simulink model "TP_EBS_CHERIF"  (R2024b)
settings: Solver=ode45  StartTime=0.0  StopTime=10  RelTol=1e-3
InitFcn:
  | Cte_TP_ABS_CHERIF
values from neighbouring files (symbols this model uses):
  d_arriere = 1.5    [Cte_TP_ABS_CHERIF.m]
  d_avant = 1.5    [Cte_TP_ABS_CHERIF.m]
  f = 0.8    [Cte_TP_ABS_CHERIF.m]
  g = 9.81    [Cte_TP_ABS_CHERIF.m]    (also in Cte_Traction.m)
  h = 0.7    [Cte_TP_ABS_CHERIF.m]
  J = 0.5    [Cte_TP_ABS_CHERIF.m]    (also in Cte_Traction.m)
  Kd = 0    [Cte_TP_ABS_CHERIF.m]
  Ki = 10    [Cte_TP_ABS_CHERIF.m]
  Kp = 100    [Cte_TP_ABS_CHERIF.m]
  L = d_avant + d_arriere    (= 3)    [Cte_TP_ABS_CHERIF.m]    (also in Cte_Traction.m = 0.0005)
  m = 1000    [Cte_TP_ABS_CHERIF.m]    (also in Cte_Traction.m = 1500)
  rRoue = 0.3    [Cte_TP_ABS_CHERIF.m]
  Ts = 0,0001    [Cte_TP_ABS_CHERIF.m]
  v0 = 27.77    [Cte_TP_ABS_CHERIF.m]
undefined symbols (not defined in the file or in its folder): DiscIntNeverNeededParam
libraries: simulink x1
settings Model: Creator=enzoc  LastModifiedBy=enzoc
settings SolverCC: ZeroCrossAlgorithm=Adaptive
settings DebuggingCC: AlgebraicLoopMsg=none  IgnoredZcDiagnostic=none

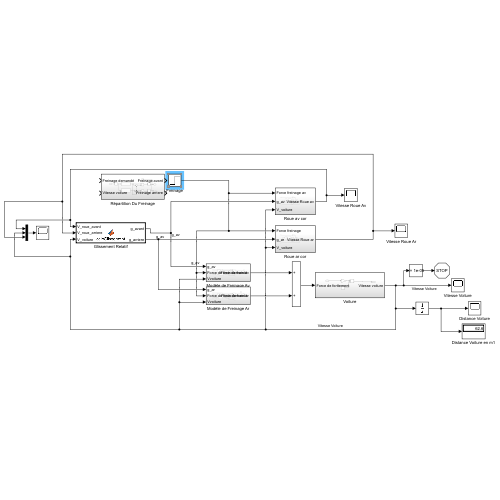
[thumbnail: Simulink's stored preview of the top-level diagram]
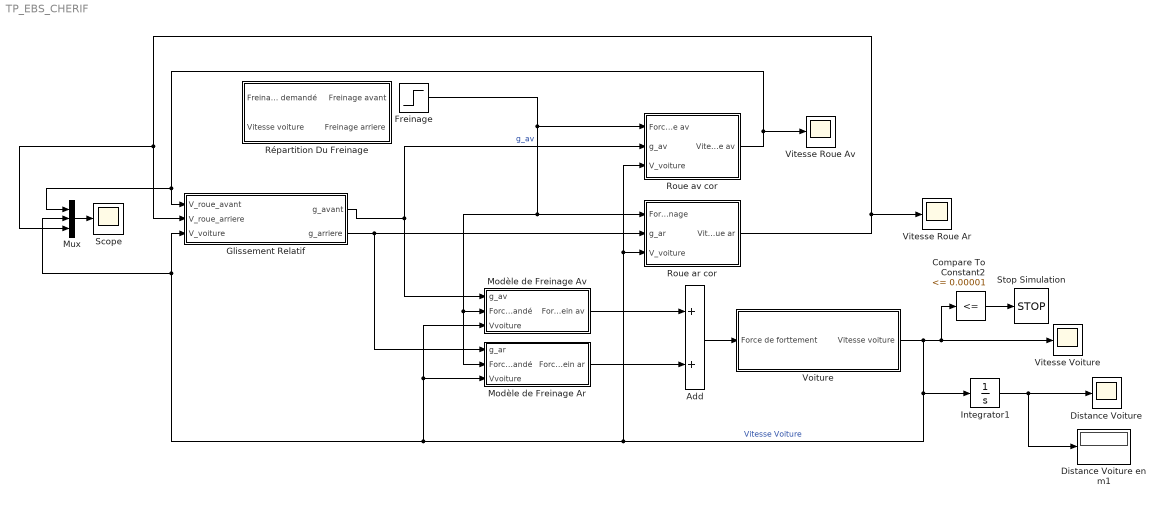
== system TP_EBS_CHERIF ==
  Add : Sum
  Compare To Constant2 : simulink/Logic and Bit Operations/Compare To Constant  relop=<=  const=0.00001  OutDataTypeStr=boolean
  Distance Voiture : Scope
  Distance Voiture en m1 : Display
  Freinage : Step  Time=0  After=4000  SampleTime=0
  Glissement Relatif : MATLAB Function  TreatAsAtomicUnit=on
  Integrator1 : Integrator
  Modèle de Freinage Ar : Subsystem
  Modèle de Freinage Av : Subsystem
  Mux : Mux  Inputs=3
  Roue ar cor : Subsystem
  Roue av cor : Subsystem
  Répartition Du Freinage : Subsystem
  Scope : Scope
  Stop Simulation : Stop
  Vitesse Roue Ar : Scope
  Vitesse Roue Av : Scope
  Vitesse Voiture : Scope
  Voiture : Subsystem
  wires:
  Glissement Relatif/1(g_avant) -> Roue av cor/2(g_av), Modèle de Freinage Av/1(g_av)  "g_av"
  Voiture/1(Vitesse voiture) -> Integrator1/1, Roue av cor/3(V_voiture), Roue ar cor/3(V_voiture), Modèle de Freinage Ar/3(Vvoiture), Modèle de Freinage Av/3(Vvoiture), Glissement Relatif/3(V_voiture), Mux/2, Compare To Constant2/1, Vitesse Voiture/1  "Vitesse Voiture"
  Modèle de Freinage Av/1(Force de frein av) -> Add/1
  Integrator1/1 -> Distance Voiture/1, Distance Voiture en m1/1
  Mux/1 -> Scope/1
  Compare To Constant2/1 -> Stop Simulation/1
  Roue av cor/1(Vitesse Roue av) -> Vitesse Roue Av/1, Mux/1, Glissement Relatif/1(V_roue_avant)
  Modèle de Freinage Ar/1(Force de frein ar) -> Add/2
  Add/1 -> Voiture/1(Force de forttement)
  Glissement Relatif/2(g_arriere) -> Roue ar cor/2(g_ar), Modèle de Freinage Ar/1(g_ar)
  Roue ar cor/1(Vitesse Roue ar) -> Mux/3, Glissement Relatif/2(V_roue_arriere), Vitesse Roue Ar/1
  Freinage/1 -> Modèle de Freinage Ar/2(Force de frein demandé), Modèle de Freinage Av/2(Force de frein demandé), Roue ar cor/1(Force freinage), Roue av cor/1(Force freinage av)

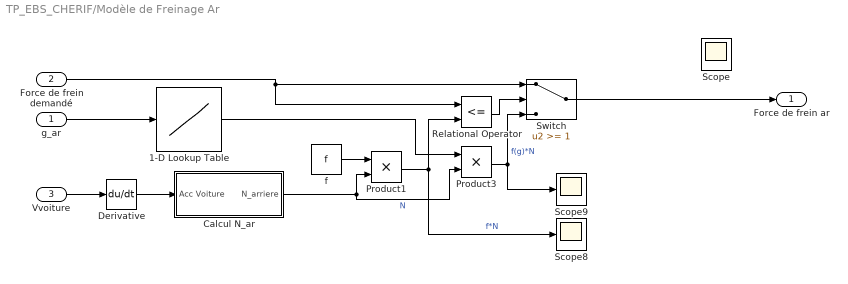
== system TP_EBS_CHERIF/Modèle de Freinage Ar ==
  g_ar : Inport
  Force de frein demandé : Inport  Port=2
  Vvoiture : Inport  Port=3
  1-D Lookup Table : Lookup_n-D  NumberOfTableDimensions=1  BreakpointsForDimension1=[0;0.050000000000000003;0.10000000000000001;0.14999999999999999;0.20000000000000001;0.25;0.29999999999999999;0.34999999999999998;0.40000000000000002;0.45000000000000001;0.5;0.55000000000000004;0.59999999999999998;0.65000000000000002;0.69999999999999996;0.75;0.80000000000000004;0.84999999999999998;0.90000000000000002;0.94999999999999996;1]  Table=[0;0.59999999999999998;0.92000000000000004;0.93999999999999995;0.94999999999999996;0.93000000000000005;0.90000000000000002;0.84999999999999998;0.80000000000000004;0.75;0.69999999999999996;0.67000000000000004;0.66000000000000003;0.65000000000000002;0.64500000000000002;0.64000000000000001;0.63700000000000001;0.63500000000000001;0.63;0.625;0.62]  InternalRulePriority=Speed  RndMeth=Simplest
  Calcul N_ar : Subsystem
  Derivative : Derivative
  Product1 : Product
  Product3 : Product
  Relational Operator : RelationalOperator  Operator=<=  OutDataTypeStr=boolean  RndMeth=Simplest  InputSameDT=off
  Scope : Scope
  Scope8 : Scope
  Scope9 : Scope
  Switch : Switch  Threshold=1  SaturateOnIntegerOverflow=off  InputSameDT=off
  f : Constant  Value=f
  Force de frein ar : Outport
  wires:
  Force de frein demandé/1 -> Relational Operator/1, Switch/1
  Product3/1 -> Scope9/1, Switch/3  "f(g)*N"
  Product1/1 -> Scope8/1, Relational Operator/2  "f*N"
  Calcul N_ar/1(N_arriere) -> Product3/2, Product1/2  "N"
  f/1 -> Product1/1
  Relational Operator/1 -> Switch/2
  g_ar/1 -> 1-D Lookup Table/1
  1-D Lookup Table/1 -> Product3/1
  Switch/1 -> Force de frein ar/1
  Vvoiture/1 -> Derivative/1
  Derivative/1 -> Calcul N_ar/1(Acc Voiture)

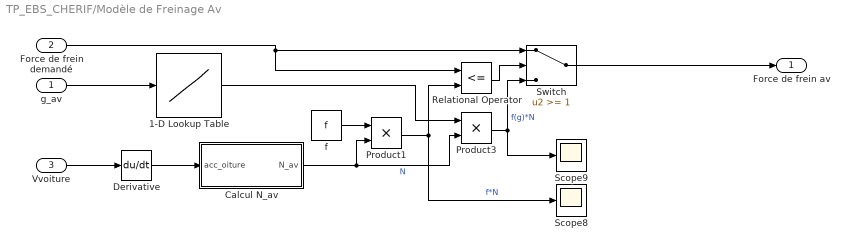
== system TP_EBS_CHERIF/Modèle de Freinage Av ==
  g_av : Inport
  Force de frein demandé : Inport  Port=2
  Vvoiture : Inport  Port=3
  1-D Lookup Table : Lookup_n-D  NumberOfTableDimensions=1  BreakpointsForDimension1=[0;0.050000000000000003;0.10000000000000001;0.14999999999999999;0.20000000000000001;0.25;0.29999999999999999;0.34999999999999998;0.40000000000000002;0.45000000000000001;0.5;0.55000000000000004;0.59999999999999998;0.65000000000000002;0.69999999999999996;0.75;0.80000000000000004;0.84999999999999998;0.90000000000000002;0.94999999999999996;1]  Table=[0;0.59999999999999998;0.92000000000000004;0.93999999999999995;0.94999999999999996;0.93000000000000005;0.90000000000000002;0.84999999999999998;0.80000000000000004;0.75;0.69999999999999996;0.67000000000000004;0.66000000000000003;0.65000000000000002;0.64500000000000002;0.64000000000000001;0.63700000000000001;0.63500000000000001;0.63;0.625;0.62]  InternalRulePriority=Speed  RndMeth=Simplest
  Calcul N_av : Subsystem
  Derivative : Derivative
  Product1 : Product
  Product3 : Product
  Relational Operator : RelationalOperator  Operator=<=  OutDataTypeStr=boolean  RndMeth=Simplest  InputSameDT=off
  Scope8 : Scope
  Scope9 : Scope
  Switch : Switch  Threshold=1  SaturateOnIntegerOverflow=off  InputSameDT=off
  f : Constant  Value=f
  Force de frein av : Outport
  wires:
  Force de frein demandé/1 -> Relational Operator/1, Switch/1
  Product3/1 -> Scope9/1, Switch/3  "f(g)*N"
  Product1/1 -> Scope8/1, Relational Operator/2  "f*N"
  Calcul N_av/1(N_av) -> Product3/2, Product1/2  "N"
  f/1 -> Product1/1
  Relational Operator/1 -> Switch/2
  g_av/1 -> 1-D Lookup Table/1
  1-D Lookup Table/1 -> Product3/1
  Switch/1 -> Force de frein av/1
  Vvoiture/1 -> Derivative/1
  Derivative/1 -> Calcul N_av/1(acc_oiture)

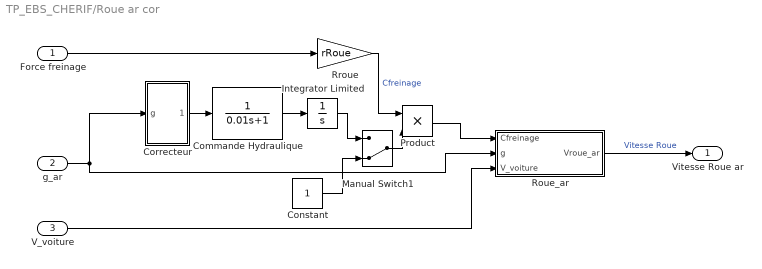
== system TP_EBS_CHERIF/Roue ar cor ==
  Force freinage : Inport
  g_ar : Inport  Port=2
  V_voiture : Inport  Port=3
  Commande Hydraulique : TransferFcn  Denominator=[0.01 1]
  Constant : Constant
  Correcteur : Subsystem
  Integrator Limited : Integrator  LimitOutput=on  UpperSaturationLimit=1000  LowerSaturationLimit=0
  Manual Switch1 : ManualSwitch  CurrentSetting=0
  Product : Product
  Roue_ar : Subsystem
  Rroue : Gain  Gain=rRoue
  Vitesse Roue ar : Outport
  wires:
  Rroue/1 -> Product/1  "Cfreinage"
  Manual Switch1/1 -> Product/2
  Correcteur/1(gcible) -> Commande Hydraulique/1
  Constant/1 -> Manual Switch1/2
  Commande Hydraulique/1 -> Integrator Limited/1
  g_ar/1 -> Roue_ar/2(g), Correcteur/1(g)
  Product/1 -> Roue_ar/1(Cfreinage)
  Integrator Limited/1 -> Manual Switch1/1
  Force freinage/1 -> Rroue/1
  Roue_ar/1(Vroue_ar) -> Vitesse Roue ar/1  "Vitesse Roue"
  V_voiture/1 -> Roue_ar/3(V_voiture)

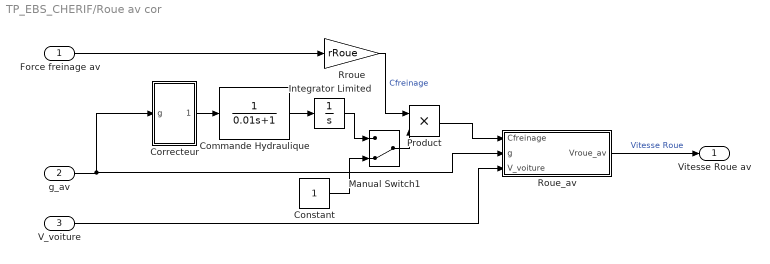
== system TP_EBS_CHERIF/Roue av cor ==
  Force freinage av : Inport
  g_av : Inport  Port=2
  V_voiture : Inport  Port=3
  Commande Hydraulique : TransferFcn  Denominator=[0.01 1]
  Constant : Constant
  Correcteur : Subsystem
  Integrator Limited : Integrator  LimitOutput=on  UpperSaturationLimit=1000  LowerSaturationLimit=0
  Manual Switch1 : ManualSwitch  CurrentSetting=0
  Product : Product
  Roue_av : Subsystem
  Rroue : Gain  Gain=rRoue
  Vitesse Roue av : Outport
  wires:
  Rroue/1 -> Product/1  "Cfreinage"
  Manual Switch1/1 -> Product/2
  Correcteur/1(gcible) -> Commande Hydraulique/1
  Constant/1 -> Manual Switch1/2
  Commande Hydraulique/1 -> Integrator Limited/1
  g_av/1 -> Correcteur/1(g), Roue_av/2(g)
  Product/1 -> Roue_av/1(Cfreinage)
  Integrator Limited/1 -> Manual Switch1/1
  Force freinage av/1 -> Rroue/1
  Roue_av/1(Vroue_av) -> Vitesse Roue av/1  "Vitesse Roue"
  V_voiture/1 -> Roue_av/3(V_voiture)

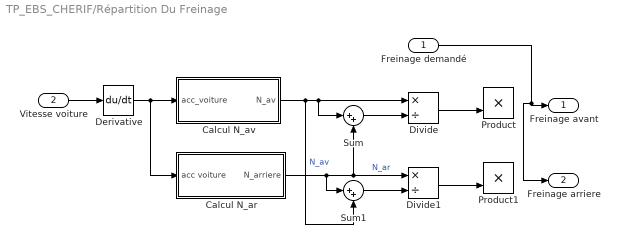
== system TP_EBS_CHERIF/Répartition Du Freinage ==
  Freinage demandé : Inport
  Vitesse voiture : Inport  Port=2
  Calcul N_ar : Subsystem
  Calcul N_av : Subsystem
  Derivative : Derivative
  Divide : Product  Inputs=*/
  Divide1 : Product  Inputs=*/
  Product : Product
  Product1 : Product
  Sum : Sum  Inputs=|++
  Sum1 : Sum  Inputs=|++
  Freinage avant : Outport
  Freinage arriere : Outport  Port=2
  wires:
  Vitesse voiture/1 -> Derivative/1
  Derivative/1 -> Calcul N_ar/1(acc voiture), Calcul N_av/1(acc_voiture)
  Calcul N_av/1(N_av) -> Sum1/2, Sum/1, Divide/1  "N_av"
  Sum/1 -> Divide/2
  Calcul N_ar/1(N_arriere) -> Sum1/1, Divide1/1, Sum/2  "N_ar"
  Sum1/1 -> Divide1/2
  Divide/1 -> Product/2
  Divide1/1 -> Product1/2
  Freinage demandé/1 -> Freinage arriere/1, Freinage avant/1

== system TP_EBS_CHERIF/Voiture ==
  Force de forttement : Inport
  -1/m : Gain  Gain=-1/m
  Integrator1 : Integrator  InitialConditionSource=external
  V : Constant  Value=v0
  Vitesse voiture : Outport
  wires:
  Force de forttement/1 -> -1/m/1
  -1/m/1 -> Integrator1/1
  Integrator1/1 -> Vitesse voiture/1
  V/1 -> Integrator1/2

== system TP_EBS_CHERIF/Modèle de Freinage Ar/Calcul N_ar ==
  Acc Voiture : Inport
  Abs : Abs  SaturateOnIntegerOverflow=off
  Add : Sum  Inputs=-+
  Constant : Constant  Value=m*g*(d_avant/L)
  Gain : Gain  Gain=m
  Gain1 : Gain  Gain=h/L
  N_arriere : Outport
  wires:
  Constant/1 -> Add/2
  Gain/1 -> Gain1/1
  Add/1 -> N_arriere/1
  Gain1/1 -> Add/1
  Abs/1 -> Gain/1
  Acc Voiture/1 -> Abs/1

== system TP_EBS_CHERIF/Modèle de Freinage Av/Calcul N_av ==
  acc_oiture : Inport
  Abs : Abs  SaturateOnIntegerOverflow=off
  Add : Sum
  Constant : Constant  Value=m*g*(d_arriere/L)
  Gain : Gain  Gain=m
  Gain1 : Gain  Gain=h/L
  N_av : Outport
  wires:
  Add/1 -> N_av/1
  Gain/1 -> Gain1/1
  Constant/1 -> Add/2
  Gain1/1 -> Add/1
  Abs/1 -> Gain/1
  acc_oiture/1 -> Abs/1

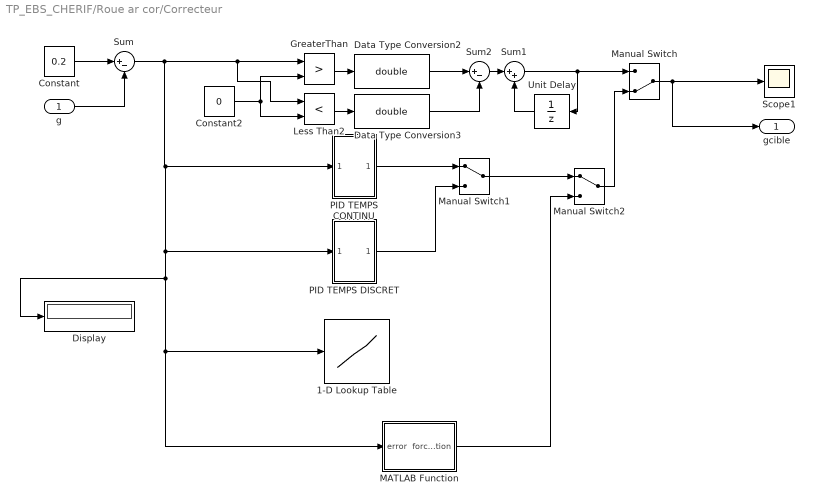
== system TP_EBS_CHERIF/Roue ar cor/Correcteur ==
  g : Inport
  1-D Lookup Table : Lookup_n-D  NumberOfTableDimensions=1  BreakpointsForDimension1=[-0.80000000000000004;-0.59999999999999998;-0.40000000000000002;-0.20000000000000001;0;0.10000000000000001;0.20000000000000001]  Table=[-800;-600;-400;-200;0;200;400]  InternalRulePriority=Speed  RndMeth=Simplest
  Constant : Constant  Value=0.2
  Constant2 : Constant  Value=0
  Data Type Conversion2 : DataTypeConversion  OutDataTypeStr=double  SaturateOnIntegerOverflow=off
  Data Type Conversion3 : DataTypeConversion  OutDataTypeStr=double  SaturateOnIntegerOverflow=off
  Display : Display
  GreaterThan : RelationalOperator  Operator=>  OutDataTypeStr=boolean  RndMeth=Simplest  InputSameDT=off
  Less Than2 : RelationalOperator  Operator=<  OutDataTypeStr=boolean  RndMeth=Simplest  InputSameDT=off
  MATLAB Function : MATLAB Function  TreatAsAtomicUnit=on
  Manual Switch : ManualSwitch  CurrentSetting=0
  Manual Switch1 : ManualSwitch
  Manual Switch2 : ManualSwitch
  PID TEMPS CONTINU : Subsystem
  PID TEMPS DISCRET : Subsystem
  Scope1 : Scope
  Sum : Sum  Inputs=|+-
  Sum1 : Sum  Inputs=|++
  Sum2 : Sum  Inputs=|+-
  Unit Delay : UnitDelay  SampleTime=0.0001  HasFrameUpgradeWarning=on
  gcible : Outport
  wires:
  Constant/1 -> Sum/1
  g/1 -> Sum/2
  GreaterThan/1 -> Data Type Conversion2/1
  Constant2/1 -> GreaterThan/2, Less Than2/2
  Data Type Conversion2/1 -> Sum2/1
  Less Than2/1 -> Data Type Conversion3/1
  Data Type Conversion3/1 -> Sum2/2
  Manual Switch/1 -> gcible/1, Scope1/1
  Sum/1 -> Display/1, MATLAB Function/1(error), 1-D Lookup Table/1, PID TEMPS DISCRET/1(In1), PID TEMPS CONTINU/1(In1), GreaterThan/1, Less Than2/1
  PID TEMPS CONTINU/1(Out1) -> Manual Switch1/1
  PID TEMPS DISCRET/1(Out1) -> Manual Switch1/2
  Sum2/1 -> Sum1/1
  Sum1/1 -> Unit Delay/1, Manual Switch/1
  Unit Delay/1 -> Sum1/2
  Manual Switch1/1 -> Manual Switch2/1
  Manual Switch2/1 -> Manual Switch/2
  MATLAB Function/1(force_correction) -> Manual Switch2/2

== system TP_EBS_CHERIF/Roue ar cor/Roue_ar ==
  Cfreinage : Inport
  g : Inport  Port=2
  V_voiture : Inport  Port=3
  Derivative : Derivative
  Gain3 : Gain  Gain=rRoue
  Subsystem : Subsystem
  Vroue_ar : Outport
  wires:
  Subsystem/1(Omega_roue_ar) -> Gain3/1
  Cfreinage/1 -> Subsystem/1(Cf)
  g/1 -> Subsystem/2(g)
  Gain3/1 -> Vroue_ar/1
  V_voiture/1 -> Derivative/1
  Derivative/1 -> Subsystem/3(acc_voiture)

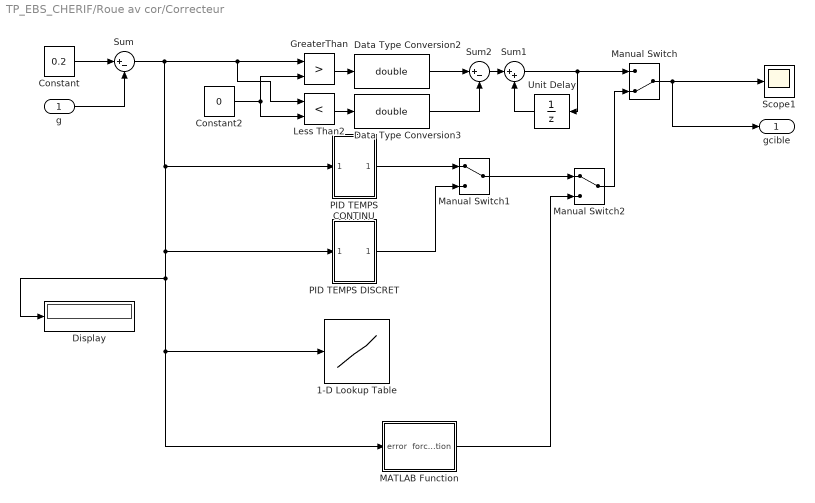
== system TP_EBS_CHERIF/Roue av cor/Correcteur ==
  g : Inport
  1-D Lookup Table : Lookup_n-D  NumberOfTableDimensions=1  BreakpointsForDimension1=[-0.80000000000000004;-0.59999999999999998;-0.40000000000000002;-0.20000000000000001;0;0.10000000000000001;0.20000000000000001]  Table=[-800;-600;-400;-200;0;200;400]  InternalRulePriority=Speed  RndMeth=Simplest
  Constant : Constant  Value=0.2
  Constant2 : Constant  Value=0
  Data Type Conversion2 : DataTypeConversion  OutDataTypeStr=double  SaturateOnIntegerOverflow=off
  Data Type Conversion3 : DataTypeConversion  OutDataTypeStr=double  SaturateOnIntegerOverflow=off
  Display : Display
  GreaterThan : RelationalOperator  Operator=>  OutDataTypeStr=boolean  RndMeth=Simplest  InputSameDT=off
  Less Than2 : RelationalOperator  Operator=<  OutDataTypeStr=boolean  RndMeth=Simplest  InputSameDT=off
  MATLAB Function : MATLAB Function  TreatAsAtomicUnit=on
  Manual Switch : ManualSwitch  CurrentSetting=0
  Manual Switch1 : ManualSwitch
  Manual Switch2 : ManualSwitch
  PID TEMPS CONTINU : Subsystem
  PID TEMPS DISCRET : Subsystem
  Scope1 : Scope
  Sum : Sum  Inputs=|+-
  Sum1 : Sum  Inputs=|++
  Sum2 : Sum  Inputs=|+-
  Unit Delay : UnitDelay  SampleTime=0.0001  HasFrameUpgradeWarning=on
  gcible : Outport
  wires:
  Constant/1 -> Sum/1
  g/1 -> Sum/2
  GreaterThan/1 -> Data Type Conversion2/1
  Constant2/1 -> GreaterThan/2, Less Than2/2
  Data Type Conversion2/1 -> Sum2/1
  Less Than2/1 -> Data Type Conversion3/1
  Data Type Conversion3/1 -> Sum2/2
  Manual Switch/1 -> gcible/1, Scope1/1
  Sum/1 -> Display/1, MATLAB Function/1(error), 1-D Lookup Table/1, PID TEMPS DISCRET/1(In1), PID TEMPS CONTINU/1(In1), GreaterThan/1, Less Than2/1
  PID TEMPS CONTINU/1(Out1) -> Manual Switch1/1
  PID TEMPS DISCRET/1(Out1) -> Manual Switch1/2
  Sum2/1 -> Sum1/1
  Sum1/1 -> Unit Delay/1, Manual Switch/1
  Unit Delay/1 -> Sum1/2
  Manual Switch1/1 -> Manual Switch2/1
  Manual Switch2/1 -> Manual Switch/2
  MATLAB Function/1(force_correction) -> Manual Switch2/2

== system TP_EBS_CHERIF/Roue av cor/Roue_av ==
  Cfreinage : Inport
  g : Inport  Port=2
  V_voiture : Inport  Port=3
  Derivative : Derivative
  Gain3 : Gain  Gain=rRoue
  Subsystem : Subsystem
  Vroue_av : Outport
  wires:
  Subsystem/1(Omega_roue_av) -> Gain3/1
  Cfreinage/1 -> Subsystem/1(Cf)
  g/1 -> Subsystem/2(g)
  Gain3/1 -> Vroue_av/1
  V_voiture/1 -> Derivative/1
  Derivative/1 -> Subsystem/3(acc_voiture)

== system TP_EBS_CHERIF/Répartition Du Freinage/Calcul N_ar ==
  acc voiture : Inport
  Abs : Abs  SaturateOnIntegerOverflow=off
  Add : Sum  Inputs=-+
  Constant : Constant  Value=m*g*(d_avant/L)
  Gain : Gain  Gain=m
  Gain1 : Gain  Gain=h/L
  N_arriere : Outport
  wires:
  Constant/1 -> Add/2
  Gain/1 -> Gain1/1
  Add/1 -> N_arriere/1
  Gain1/1 -> Add/1
  Abs/1 -> Gain/1
  acc voiture/1 -> Abs/1

== system TP_EBS_CHERIF/Répartition Du Freinage/Calcul N_av ==
  acc_voiture : Inport
  Abs : Abs  SaturateOnIntegerOverflow=off
  Add : Sum
  Constant : Constant  Value=m*g*(d_arriere/L)
  Gain : Gain  Gain=m
  Gain1 : Gain  Gain=h/L
  N_av : Outport
  wires:
  Add/1 -> N_av/1
  Gain/1 -> Gain1/1
  Constant/1 -> Add/2
  Gain1/1 -> Add/1
  Abs/1 -> Gain/1
  acc_voiture/1 -> Abs/1

== system TP_EBS_CHERIF/Roue ar cor/Correcteur/PID TEMPS CONTINU ==
  In1 : Inport
  Add : Sum  Inputs=+++
  Derivative : Derivative
  Gain : Gain  Gain=Kp
  Gain1 : Gain  Gain=Ki
  Gain2 : Gain  Gain=Kd
  Integrator : Integrator
  Out1 : Outport
  wires:
  Derivative/1 -> Add/3
  Add/1 -> Out1/1
  In1/1 -> Gain2/1, Gain1/1, Gain/1
  Gain/1 -> Add/1
  Gain2/1 -> Derivative/1
  Integrator/1 -> Add/2
  Gain1/1 -> Integrator/1

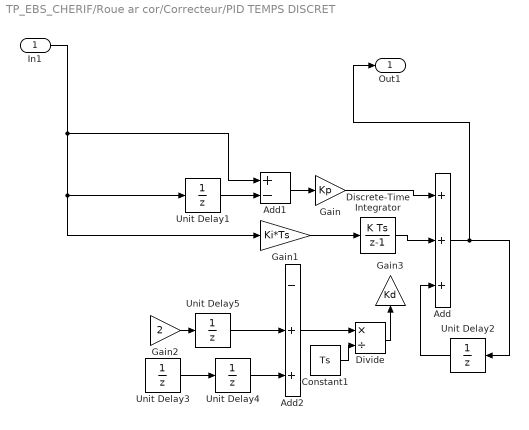
== system TP_EBS_CHERIF/Roue ar cor/Correcteur/PID TEMPS DISCRET ==
  In1 : Inport
  Add : Sum  Inputs=+++
  Add1 : Sum  Inputs=+-
  Add2 : Sum  Inputs=-++
  Constant1 : Constant  Value=Ts
  Discrete-Time Integrator : DiscreteIntegrator  SampleTime=-1  ICPrevOutput=DiscIntNeverNeededParam  ICPrevScaledInput=DiscIntNeverNeededParam
  Divide : Product  Inputs=*/
  Gain : Gain  Gain=Kp
  Gain1 : Gain  Gain=Ki*Ts
  Gain2 : Gain  Gain=2
  Gain3 : Gain  Gain=Kd
  Unit Delay{1..5} (5 alike) : UnitDelay  SampleTime=0.0001  HasFrameUpgradeWarning=on
  Out1 : Outport
  wires:
  In1/1 -> Gain1/1, Unit Delay1/1, Add1/1
  Gain2/1 -> Unit Delay5/1
  Add/1 -> Out1/1, Unit Delay2/1
  Constant1/1 -> Divide/2
  Divide/1 -> Gain3/1
  Unit Delay4/1 -> Add2/3
  Unit Delay5/1 -> Add2/2
  Add2/1 -> Divide/1
  Unit Delay3/1 -> Unit Delay4/1
  Gain1/1 -> Discrete-Time Integrator/1
  Unit Delay1/1 -> Add1/2
  Gain/1 -> Add/1
  Discrete-Time Integrator/1 -> Add/2
  Add1/1 -> Gain/1
  Unit Delay2/1 -> Add/3

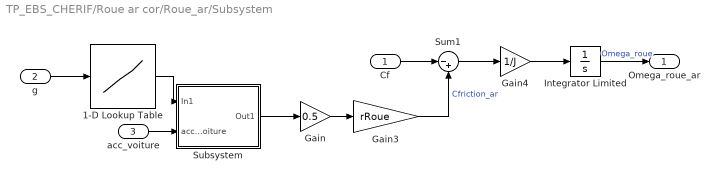
== system TP_EBS_CHERIF/Roue ar cor/Roue_ar/Subsystem ==
  Cf : Inport
  g : Inport  Port=2
  acc_voiture : Inport  Port=3
  1-D Lookup Table : Lookup_n-D  NumberOfTableDimensions=1  BreakpointsForDimension1=[0;0.050000000000000003;0.10000000000000001;0.14999999999999999;0.20000000000000001;0.25;0.29999999999999999;0.34999999999999998;0.40000000000000002;0.45000000000000001;0.5;0.55000000000000004;0.59999999999999998;0.65000000000000002;0.69999999999999996;0.75;0.80000000000000004;0.84999999999999998;0.90000000000000002;0.94999999999999996;1]  Table=[0;0.59999999999999998;0.92000000000000004;0.93999999999999995;0.94999999999999996;0.93000000000000005;0.90000000000000002;0.84999999999999998;0.80000000000000004;0.75;0.69999999999999996;0.67000000000000004;0.66000000000000003;0.65000000000000002;0.64500000000000002;0.64000000000000001;0.63700000000000001;0.63500000000000001;0.63;0.625;0.62]  InternalRulePriority=Speed  RndMeth=Simplest
  Gain : Gain  Gain=0.5
  Gain3 : Gain  Gain=rRoue
  Gain4 : Gain  Gain=1/J
  Integrator Limited : Integrator  InitialCondition=v0/rRoue  LimitOutput=on  UpperSaturationLimit=1000  LowerSaturationLimit=0
  Subsystem : Subsystem
  Sum1 : Sum  Inputs=|-+
  Omega_roue_ar : Outport
  wires:
  Gain/1 -> Gain3/1
  g/1 -> 1-D Lookup Table/1
  Sum1/1 -> Gain4/1
  1-D Lookup Table/1 -> Subsystem/1(In1)
  Gain4/1 -> Integrator Limited/1
  acc_voiture/1 -> Subsystem/2(acc_voiture)
  Subsystem/1(Out1) -> Gain/1
  Cf/1 -> Sum1/1
  Gain3/1 -> Sum1/2  "Cfriction_ar"
  Integrator Limited/1 -> Omega_roue_ar/1  "Omega_roue"

== system TP_EBS_CHERIF/Roue av cor/Correcteur/PID TEMPS CONTINU ==
  In1 : Inport
  Add : Sum  Inputs=+++
  Derivative : Derivative
  Gain : Gain  Gain=Kp
  Gain1 : Gain  Gain=Ki
  Gain2 : Gain  Gain=Kd
  Integrator : Integrator
  Out1 : Outport
  wires:
  Derivative/1 -> Add/3
  Add/1 -> Out1/1
  In1/1 -> Gain2/1, Gain1/1, Gain/1
  Gain/1 -> Add/1
  Gain2/1 -> Derivative/1
  Integrator/1 -> Add/2
  Gain1/1 -> Integrator/1

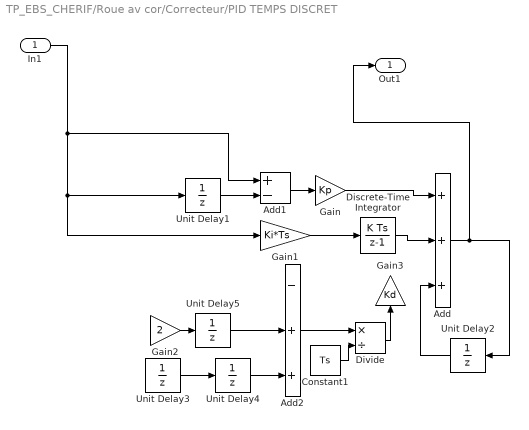
== system TP_EBS_CHERIF/Roue av cor/Correcteur/PID TEMPS DISCRET ==
  In1 : Inport
  Add : Sum  Inputs=+++
  Add1 : Sum  Inputs=+-
  Add2 : Sum  Inputs=-++
  Constant1 : Constant  Value=Ts
  Discrete-Time Integrator : DiscreteIntegrator  SampleTime=-1  ICPrevOutput=DiscIntNeverNeededParam  ICPrevScaledInput=DiscIntNeverNeededParam
  Divide : Product  Inputs=*/
  Gain : Gain  Gain=Kp
  Gain1 : Gain  Gain=Ki*Ts
  Gain2 : Gain  Gain=2
  Gain3 : Gain  Gain=Kd
  Unit Delay{1..5} (5 alike) : UnitDelay  SampleTime=0.0001  HasFrameUpgradeWarning=on
  Out1 : Outport
  wires:
  In1/1 -> Gain1/1, Unit Delay1/1, Add1/1
  Gain2/1 -> Unit Delay5/1
  Add/1 -> Out1/1, Unit Delay2/1
  Constant1/1 -> Divide/2
  Divide/1 -> Gain3/1
  Unit Delay4/1 -> Add2/3
  Unit Delay5/1 -> Add2/2
  Add2/1 -> Divide/1
  Unit Delay3/1 -> Unit Delay4/1
  Gain1/1 -> Discrete-Time Integrator/1
  Unit Delay1/1 -> Add1/2
  Gain/1 -> Add/1
  Discrete-Time Integrator/1 -> Add/2
  Add1/1 -> Gain/1
  Unit Delay2/1 -> Add/3

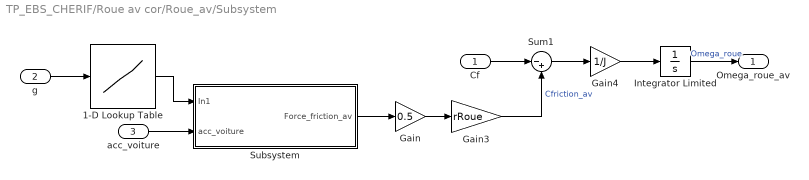
== system TP_EBS_CHERIF/Roue av cor/Roue_av/Subsystem ==
  Cf : Inport
  g : Inport  Port=2
  acc_voiture : Inport  Port=3
  1-D Lookup Table : Lookup_n-D  NumberOfTableDimensions=1  BreakpointsForDimension1=[0;0.050000000000000003;0.10000000000000001;0.14999999999999999;0.20000000000000001;0.25;0.29999999999999999;0.34999999999999998;0.40000000000000002;0.45000000000000001;0.5;0.55000000000000004;0.59999999999999998;0.65000000000000002;0.69999999999999996;0.75;0.80000000000000004;0.84999999999999998;0.90000000000000002;0.94999999999999996;1]  Table=[0;0.59999999999999998;0.92000000000000004;0.93999999999999995;0.94999999999999996;0.93000000000000005;0.90000000000000002;0.84999999999999998;0.80000000000000004;0.75;0.69999999999999996;0.67000000000000004;0.66000000000000003;0.65000000000000002;0.64500000000000002;0.64000000000000001;0.63700000000000001;0.63500000000000001;0.63;0.625;0.62]  InternalRulePriority=Speed  RndMeth=Simplest
  Gain : Gain  Gain=0.5
  Gain3 : Gain  Gain=rRoue
  Gain4 : Gain  Gain=1/J
  Integrator Limited : Integrator  InitialCondition=v0/rRoue  LimitOutput=on  UpperSaturationLimit=1000  LowerSaturationLimit=0
  Subsystem : Subsystem
  Sum1 : Sum  Inputs=|-+
  Omega_roue_av : Outport
  wires:
  Cf/1 -> Sum1/1
  g/1 -> 1-D Lookup Table/1
  Sum1/1 -> Gain4/1
  Gain3/1 -> Sum1/2  "Cfriction_av"
  1-D Lookup Table/1 -> Subsystem/1(In1)
  acc_voiture/1 -> Subsystem/2(acc_voiture)
  Subsystem/1(Force_friction_av) -> Gain/1
  Gain/1 -> Gain3/1
  Gain4/1 -> Integrator Limited/1
  Integrator Limited/1 -> Omega_roue_av/1  "Omega_roue"

== system TP_EBS_CHERIF/Roue ar cor/Roue_ar/Subsystem/Subsystem ==
  In1 : Inport
  acc_voiture : Inport  Port=2
  Abs : Abs  SaturateOnIntegerOverflow=off
  Add : Sum  Inputs=-+
  Constant : Constant  Value=m*g*(d_avant/L)
  Gain : Gain  Gain=m
  Gain1 : Gain  Gain=h/L
  Product : Product
  Out1 : Outport
  wires:
  acc_voiture/1 -> Abs/1
  Gain1/1 -> Add/1
  Gain/1 -> Gain1/1
  Constant/1 -> Add/2
  Add/1 -> Product/2
  In1/1 -> Product/1
  Product/1 -> Out1/1
  Abs/1 -> Gain/1

== system TP_EBS_CHERIF/Roue av cor/Roue_av/Subsystem/Subsystem ==
  In1 : Inport
  acc_voiture : Inport  Port=2
  Abs : Abs  SaturateOnIntegerOverflow=off
  Add : Sum
  Constant : Constant  Value=m*g*(d_arriere/L)
  Gain : Gain  Gain=m
  Gain1 : Gain  Gain=h/L
  Product : Product
  Force_friction_av : Outport
  wires:
  Constant/1 -> Add/2
  Gain/1 -> Gain1/1
  Add/1 -> Product/2
  Gain1/1 -> Add/1
  Product/1 -> Force_friction_av/1
  In1/1 -> Product/1
  acc_voiture/1 -> Abs/1
  Abs/1 -> Gain/1

== matlab function TP_EBS_CHERIF/Roue av cor/Correcteur/MATLAB Function ==
  settings: updateMethod=DISCRETE
  data: error input; force_correction output
function force_correction = ABS_Control(error)
    % Définir les limites de la force de freinage
    max_force = 800;
    min_force = -800;

    % Initialiser la force de correction
    persistent current_force
    if isempty(current_force)
        current_force = 0;  % Valeur initiale de la force de freinage
    end

    % Ajustement de la force en fonction de l'erreur
    if error > 0.05
        % Si l'erreur est positive, augmenter la force de freinage
        current_force = current_force + 100;
    elseif error < -0.05
        % Si l'erreur est négative, diminuer la force de freinage
        current_force = current_force - 100;
    end

    % Appliquer les limites de saturation
    if current_force > max_force
        current_force = max_force;
    elseif current_force < min_force
        current_force = min_force;
    end

    % Sortie de la fonction
    force_correction = current_force;
end

== matlab function TP_EBS_CHERIF/Glissement Relatif ==
  data: V_roue_avant input; V_roue_arriere input; V_voiture input; g_avant output; g_arriere output
function [g_avant, g_arriere] = calcGlissement(V_roue_avant, V_roue_arriere, V_voiture)
    % Calcul du glissement pour le train avant
    g_avant = 1 - (V_roue_avant / V_voiture);
    
    % Calcul du glissement pour le train arrière
    g_arriere = 1 - (V_roue_arriere / V_voiture);
end

== matlab function TP_EBS_CHERIF/Roue ar cor/Correcteur/MATLAB Function ==
  settings: updateMethod=DISCRETE
  data: error input; force_correction output
function force_correction = ABS_Control(error)
    % Définir les limites de la force de freinage
    max_force = 800;
    min_force = -800;

    % Initialiser la force de correction
    persistent current_force
    if isempty(current_force)
        current_force = 0;  % Valeur initiale de la force de freinage
    end

    % Ajustement de la force en fonction de l'erreur
    if error > 0.05
        % Si l'erreur est positive, augmenter la force de freinage
        current_force = current_force + 100;
    elseif error < -0.05
        % Si l'erreur est négative, diminuer la force de freinage
        current_force = current_force - 100;
    end

    % Appliquer les limites de saturation
    if current_force > max_force
        current_force = max_force;
    elseif current_force < min_force
        current_force = min_force;
    end

    % Sortie de la fonction
    force_correction = current_force;
end
